simulink model "sampleModel1770"  (R2023a)
settings: Solver=VariableStepAuto  StartTime=0.0  StopTime=10.0  RelTol=1e-3
libraries: simulink x6, hdlsllib x4
settings Model: Creator=user1  LastModifiedBy=user1

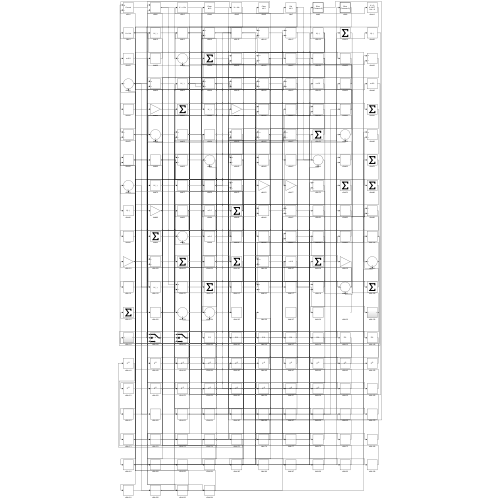
[thumbnail: Simulink's stored preview of the top-level diagram]
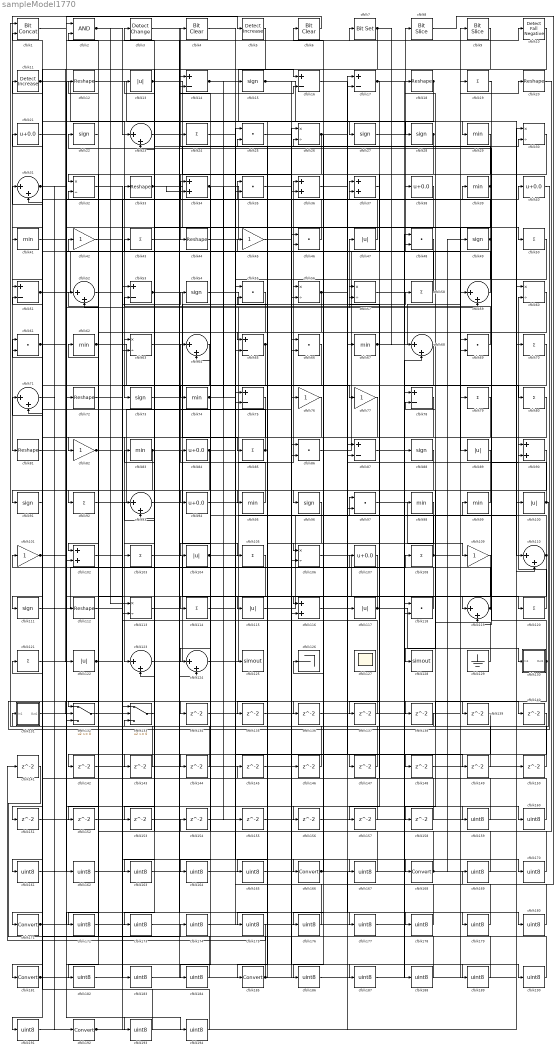
== system sampleModel1770 ==
  cfblk1 : hdlsllib/Logic and Bit Operations/Bit Concat  numInputs=2
  cfblk10 : hdlsllib/Logic and Bit Operations/Detect Fall Negative  vinit=0  OutDataTypeStr=boolean
  cfblk{13,47,89,100,104,115,117,122} (8 alike) : Abs  SaturateOnIntegerOverflow=off
  cfblk{42,45,76..77,82,101,109} (7 alike) : Gain
  cfblk{34,36..37,90,102,116} (6 alike) : Sum
  cfblk{19,24,43,50,58,70,79..80,85,92,103,105,108,114,120..121} (16 alike) : Sum  Inputs=+
  cfblk{26,30,32,56..57,60,63,106,113} (9 alike) : Product  Inputs=*/  RndMeth=Zero  SaturateOnIntegerOverflow=on
  cfblk{21,38,40,84,94,107} (6 alike) : Bias  Bias=0.0  SaturateOnIntegerOverflow=off
  cfblk11 : simulink/Logic and Bit Operations/Detect Increase  vinit=0.0  OutDataTypeStr=boolean
      settings: LibrarySourceBlock=|
      | hdlsllib/Logic and Bit
      | Operations/Detect
      | Increase
  cfblk{23,31,52,59,64,68,71,93,110,119,123..124} (12 alike) : Sum  Inputs=|++
  cfblk{15,22,27..28,49,54,73,88,91,96,111} (11 alike) : Signum
  cfblk{12,18,20,33,44,72,81,112} (8 alike) : Reshape
  cfblk{25,35,46,48,55,61,66,69,86,97,118} (11 alike) : DotProduct  OutDataTypeStr=Inherit: Inherit via internal rule
  cfblk125 : ToWorkspace  VariableName=simout  SaveFormat=Timeseries  SampleTime=-1
  cfblk126 : Terminator
  cfblk127 : Scope
      settings: Floating=on
  cfblk128 : ToWorkspace  VariableName=simout  SaveFormat=Timeseries  SampleTime=-1
  cfblk129 : Ground
  cfblk130 : Subsystem
      settings: LibrarySourceBlock=|
      | hdlsllib/Ports &
      | Subsystems/Subsystem
  cfblk131 : Subsystem
      settings: LibrarySourceBlock=|
      | hdlsllib/Ports &
      | Subsystems/Subsystem
  cfblk132 : Switch  SaturateOnIntegerOverflow=off  InputSameDT=off
  cfblk133 : Switch  SaturateOnIntegerOverflow=off  InputSameDT=off
  cfblk{134..158} (25 alike) : Delay  SampleTime=1
  cfblk{14,16..17,51,53,65,75,78,87} (9 alike) : Sum  Inputs=+-
  cfblk{159..165,167,169..170,172..180,182..184,186..191,193..194} (30 alike) : DataTypeConversion  OutDataTypeStr=uint8  SaturateOnIntegerOverflow=off  RndMeth=Floor
  cfblk{166,168,171,181,185,192} (6 alike) : DataTypeConversion  SaturateOnIntegerOverflow=off  RndMeth=Floor
  cfblk2 : Logic  AllPortsSameDT=off  OutDataTypeStr=boolean
  cfblk{29,39,41,62,67,74,83,95,98..99} (10 alike) : MinMax
  cfblk3 : simulink/Logic and Bit Operations/Detect Change  vinit=0  OutDataTypeStr=boolean
      settings: LibrarySourceBlock=|
      | hdlsllib/Logic and Bit
      | Operations/Detect
      | Change
  cfblk4 : simulink/Logic and Bit Operations/Bit Clear  iBit=0
      settings: LibrarySourceBlock=|
      | hdlsllib/Logic and Bit
      | Operations/Bit Clear
  cfblk5 : simulink/Logic and Bit Operations/Detect Increase  vinit=0.0  OutDataTypeStr=boolean
      settings: LibrarySourceBlock=|
      | hdlsllib/Logic and Bit
      | Operations/Detect
      | Increase
  cfblk6 : simulink/Logic and Bit Operations/Bit Clear  iBit=0
      settings: LibrarySourceBlock=|
      | hdlsllib/Logic and Bit
      | Operations/Bit Clear
  cfblk7 : simulink/Logic and Bit Operations/Bit Set  iBit=0
      settings: LibrarySourceBlock=|
      | hdlsllib/Logic and Bit
      | Operations/Bit Set
  cfblk8 : hdlsllib/Logic and Bit Operations/Bit Slice  lidx=7  ridx=0
  cfblk9 : hdlsllib/Logic and Bit Operations/Bit Slice  lidx=7  ridx=0
  wires:
  cfblk130/1(Out1) -> cfblk22/1, cfblk158/1
  cfblk9/1 -> cfblk122/1
  cfblk124/1 -> cfblk47/1
  cfblk53/1 -> cfblk85/1, cfblk16/2
  cfblk94/1 -> cfblk36/1
  cfblk39/1 -> cfblk4/1, cfblk124/1, cfblk13/1
  cfblk58/1 -> cfblk32/1
  cfblk79/1 -> cfblk185/1
  cfblk65/1 -> cfblk95/1, cfblk151/1
  cfblk104/1 -> cfblk99/1, cfblk57/2
  cfblk11/1 -> cfblk73/1, cfblk138/1
  cfblk110/1 -> cfblk97/1, cfblk116/1
  cfblk44/1 -> cfblk37/1
  cfblk103/1 -> cfblk119/1
  cfblk24/1 -> cfblk166/1
  cfblk86/1 -> cfblk8/1
  cfblk97/1 -> cfblk109/1
  cfblk83/1 -> cfblk105/1, cfblk111/1
  cfblk54/1 -> cfblk58/1
  cfblk17/1 -> cfblk118/1, cfblk157/1
  cfblk13/1 -> cfblk36/2, cfblk124/2
  cfblk14/1 -> cfblk29/1, cfblk16/1
  cfblk99/1 -> cfblk92/1
  cfblk18/1 -> cfblk65/1, cfblk51/1, cfblk153/1
  cfblk23/1 -> cfblk27/1
  cfblk75/1 -> cfblk171/1
  cfblk108/1 -> cfblk20/1, cfblk64/2
  cfblk78/1 -> cfblk123/1
  cfblk92/1 -> cfblk26/1
  cfblk36/1 -> cfblk67/1
  cfblk6/1 -> cfblk81/1
  cfblk120/1 -> cfblk60/2
  cfblk29/1 -> cfblk102/1
  cfblk123/1 -> cfblk56/1
  cfblk60/1 -> cfblk82/1
  cfblk30/1 -> cfblk44/1
  cfblk15/1 -> cfblk28/1, cfblk148/1
  cfblk67/1 -> cfblk48/1, cfblk19/1
  cfblk41/1 -> cfblk50/1
  cfblk33/1 -> cfblk17/1, cfblk89/1, cfblk34/2
  cfblk85/1 -> cfblk33/1, cfblk51/2
  cfblk88/1 -> cfblk181/1
  cfblk93/1 -> cfblk168/1
  cfblk69/1 -> cfblk53/2
  cfblk89/1 -> cfblk132/1
  cfblk100/1 -> cfblk131/1(In1), cfblk39/1
  cfblk82/1 -> cfblk12/1, cfblk52/1, cfblk40/1
  cfblk122/1 -> cfblk108/1, cfblk34/1
  cfblk133/1 -> cfblk43/1
  cfblk49/1 -> cfblk14/1, cfblk65/2, cfblk18/1
  cfblk61/1 -> cfblk113/2, cfblk193/1
  cfblk38/1 -> cfblk103/1
  cfblk34/1 -> cfblk37/2, cfblk94/1, cfblk155/1
  cfblk95/1 -> cfblk64/1
  cfblk111/1 -> cfblk14/2
  cfblk117/1 -> cfblk130/1(In1), cfblk115/1, cfblk90/2
  cfblk66/1 -> cfblk91/1
  cfblk40/1 -> cfblk132/2
  cfblk129/1 -> cfblk38/1
  cfblk43/1 -> cfblk10/1
  cfblk84/1 -> cfblk48/2, cfblk142/1
  cfblk56/1 -> cfblk117/1, cfblk104/1
  cfblk106/1 -> cfblk120/1
  cfblk81/1 -> cfblk35/1
  cfblk2/1 -> cfblk23/1, cfblk113/1
  cfblk119/1 -> cfblk83/1, cfblk57/1
  cfblk90/1 -> cfblk128/1
  cfblk22/1 -> cfblk2/2
  cfblk51/1 -> cfblk9/1, cfblk194/1
  cfblk68/1 -> cfblk102/2
  cfblk32/1 -> cfblk74/1
  cfblk1/1 -> cfblk5/1
  cfblk118/1 -> cfblk101/1
  cfblk26/1 -> cfblk96/1, cfblk52/2, cfblk30/2
  cfblk12/1 -> cfblk110/1
  cfblk131/1(Out1) -> cfblk46/2
  cfblk27/1 -> cfblk80/1
  cfblk115/1 -> cfblk30/1
  cfblk7/1 -> cfblk41/1, cfblk35/2, cfblk68/1
  cfblk101/1 -> cfblk59/2, cfblk162/1
  cfblk74/1 -> cfblk125/1, cfblk15/1
  cfblk62/1 -> cfblk77/1, cfblk116/2
  cfblk73/1 -> cfblk26/2
  cfblk46/1 -> cfblk11/1
  cfblk28/1 -> cfblk63/1, cfblk186/1
  cfblk50/1 -> cfblk106/1
  cfblk107/1 -> cfblk114/1
  cfblk91/1 -> cfblk61/1
  cfblk47/1 -> cfblk21/1
  cfblk35/1 -> cfblk76/1
  cfblk102/1 -> cfblk54/1
  cfblk71/1 -> cfblk192/1
  cfblk116/1 -> cfblk90/1
  cfblk59/1 -> cfblk31/2
  cfblk19/1 -> cfblk119/2
  cfblk21/1 -> cfblk132/3
  cfblk31/1 -> cfblk7/1, cfblk112/1, cfblk156/1
  cfblk72/1 -> cfblk134/1
  cfblk134/1 -> cfblk69/2
  cfblk96/1 -> cfblk135/1
  cfblk52/1 -> cfblk136/1
  cfblk136/1 -> cfblk17/2
  cfblk37/1 -> cfblk137/1
  cfblk137/1 -> cfblk53/1
  cfblk138/1 -> cfblk133/3
  cfblk4/1 -> cfblk139/1
  cfblk132/1 -> cfblk140/1
  cfblk142/1 -> cfblk56/2
  cfblk77/1 -> cfblk143/1
  cfblk143/1 -> cfblk1/1
  cfblk76/1 -> cfblk144/1
  cfblk144/1 -> cfblk2/1
  cfblk145/1 -> cfblk66/2
  cfblk146/1 -> cfblk61/2
  cfblk114/1 -> cfblk147/1
  cfblk147/1 -> cfblk31/1
  cfblk148/1 -> cfblk110/2
  cfblk16/1 -> cfblk149/1
  cfblk149/1 -> cfblk78/2
  cfblk150/1 -> cfblk23/2
  cfblk151/1 -> cfblk133/1
  cfblk64/1 -> cfblk152/1
  cfblk152/1 -> cfblk60/1
  cfblk153/1 -> cfblk86/1
  cfblk20/1 -> cfblk154/1
  cfblk154/1 -> cfblk59/1
  cfblk155/1 -> cfblk106/2
  cfblk156/1 -> cfblk118/2
  cfblk157/1 -> cfblk123/2
  cfblk158/1 -> cfblk1/2
  cfblk3/1 -> cfblk159/1
  cfblk159/1 -> cfblk107/1
  cfblk63/1 -> cfblk160/1
  cfblk160/1 -> cfblk3/1
  cfblk70/1 -> cfblk161/1
  cfblk161/1 -> cfblk72/1
  cfblk162/1 -> cfblk70/1
  cfblk55/1 -> cfblk163/1
  cfblk163/1 -> cfblk69/1
  cfblk140/1 -> cfblk164/1
  cfblk164/1 -> cfblk55/1
  cfblk80/1 -> cfblk165/1
  cfblk165/1 -> cfblk55/2
  cfblk166/1 -> cfblk126/1, cfblk6/1, cfblk180/1
  cfblk45/1 -> cfblk167/1
  cfblk167/1 -> cfblk24/1
  cfblk168/1 -> cfblk32/2, cfblk49/1
  cfblk8/1 -> cfblk169/1
  cfblk169/1 -> cfblk93/1
  cfblk112/1 -> cfblk170/1
  cfblk170/1 -> cfblk93/2
  cfblk171/1 -> cfblk78/1, cfblk179/1
  cfblk139/1 -> cfblk172/1
  cfblk172/1 -> cfblk75/1
  cfblk10/1 -> cfblk173/1
  cfblk173/1 -> cfblk75/2
  cfblk141/1 -> cfblk174/1
  cfblk174/1 -> cfblk97/2
  cfblk48/1 -> cfblk175/1
  cfblk175/1 -> cfblk141/1
  cfblk98/1 -> cfblk176/1
  cfblk176/1 -> cfblk46/1
  cfblk113/1 -> cfblk177/1
  cfblk177/1 -> cfblk98/1
  cfblk25/1 -> cfblk178/1
  cfblk178/1 -> cfblk145/1
  cfblk179/1 -> cfblk25/1
  cfblk180/1 -> cfblk25/2
  cfblk181/1 -> cfblk68/2, cfblk86/2, cfblk66/1
  cfblk109/1 -> cfblk182/1
  cfblk182/1 -> cfblk88/1
  cfblk42/1 -> cfblk183/1
  cfblk183/1 -> cfblk84/1
  cfblk105/1 -> cfblk184/1
  cfblk184/1 -> cfblk42/1
  cfblk185/1 -> cfblk146/1, cfblk45/1, cfblk62/1
  cfblk186/1 -> cfblk79/1
  cfblk121/1 -> cfblk187/1
  cfblk187/1 -> cfblk150/1
  cfblk57/1 -> cfblk188/1
  cfblk188/1 -> cfblk121/1
  cfblk87/1 -> cfblk189/1
  cfblk189/1 -> cfblk133/2
  cfblk135/1 -> cfblk190/1
  cfblk190/1 -> cfblk87/1
  cfblk5/1 -> cfblk191/1
  cfblk191/1 -> cfblk87/2
  cfblk192/1 -> cfblk63/2, cfblk100/1
  cfblk193/1 -> cfblk71/1
  cfblk194/1 -> cfblk71/2

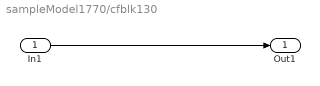
== system sampleModel1770/cfblk130 ==
  In1 : Inport
  Out1 : Outport
  wires:
  In1/1 -> Out1/1

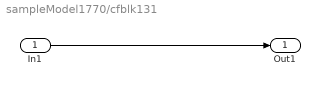
== system sampleModel1770/cfblk131 ==
  In1 : Inport
  Out1 : Outport
  wires:
  In1/1 -> Out1/1
